simulink subsystem "tof_sensors"  (R2022b)
settings: Solver=VariableStepAuto  StartTime=0.0  StopTime=10.0  RelTol=1e-3
model mask{Pin=D5}
  mask prompts: Pin "Sync Pin"
undefined symbols (not defined in the file): t_step
libraries: mbedblockslib x2
settings Model: Creator=micha  LastModifiedBy=micha

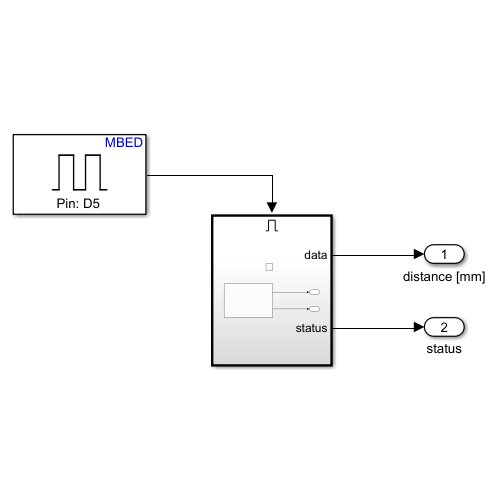
[thumbnail: Simulink's stored preview of the top-level diagram]
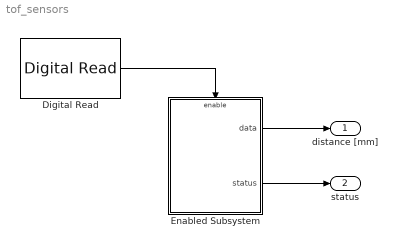
== system tof_sensors ==
  Digital Read : mbedblockslib/Digital Read  Pin=D5  Direction=input  SampleTime=-1
      settings: LibrarySourceBlock=stmnucleorootlib/Common/Digital Read
  Enabled Subsystem : Subsystem  TreatAsAtomicUnit=on
  distance [mm] : Outport
  status : Outport  Port=2
  wires:
  Digital Read/1 -> Enabled Subsystem/Enable
  Enabled Subsystem/1(data) -> distance [mm]/1
  Enabled Subsystem/2(status) -> status/1

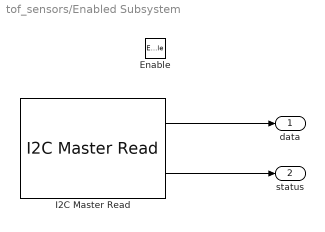
== system tof_sensors/Enabled Subsystem ==
  Enable : EnablePort
  I2C Master Read : mbedblockslib/I2C Master Read  I2CModule=2  Mode=Master  SlaveAddress=hex2dec('02')  SlaveByteOrder=BigEndian  Direction=Receiver  RegisterAddressMode=off  RegisterAddress=uint8(1)  SlaveDataType=uint16  DataLength=2  NoAck=off  RepeatedStart=off  OutputStatus=on  SampleTime=t_step
      settings: LibrarySourceBlock=stmnucleorootlib/Common/I2C Master Read
  data : Outport
  status : Outport  Port=2
  wires:
  I2C Master Read/2 -> status/1
  I2C Master Read/1 -> data/1
